simulink model "holo"  (R2012b)
settings: Solver=FixedStepDiscrete  SolverMode=SingleTasking  StartTime=0.0  StopTime=160000  RelTol=1e-3
undefined symbols (not defined in the file): xlipgetpartsetting
libraries: xbsIndex_r4 x3259, casper_library_misc x36, simulink x18, dspsigops x12, casper_library_delays x8, xps_library x5, casper_library_multipliers x4
(part 5 of 34)

== system holo/dec_fir1 ==
  sync_in : Inport
  real1 : Inport  Port=2
  imag1 : Inport  Port=3
  real2 : Inport  Port=4
  imag2 : Inport  Port=5
  real3 : Inport  Port=6
  imag3 : Inport  Port=7
  real4 : Inport  Port=8
  imag4 : Inport  Port=9
  convert1 : xbsIndex_r4/Convert  gui_display_data_type=Fixed-point  arith_type="Signed  (2's comp)"  n_bits=25  bin_pt=24  float_type=Single  exp_bits=8  fraction_bits=24  quantization="Round  (unbiased: +/- Inf)"  overflow=Wrap  en=off  latency=2  dbl_ovrd=off  pipeline=off  block_type=convert
  convert2 : xbsIndex_r4/Convert  gui_display_data_type=Fixed-point  arith_type="Signed  (2's comp)"  n_bits=25  bin_pt=24  float_type=Single  exp_bits=8  fraction_bits=24  quantization="Round  (unbiased: +/- Inf)"  overflow=Wrap  en=off  latency=2  dbl_ovrd=off  pipeline=off  block_type=convert
  delay : xbsIndex_r4/Delay  rst=off  infoeditControl=Selection of Reset will increase slice count due to use of real FFs and instead of SRLs  en=off  latency=7  dbl_ovrd=off  reg_retiming=off  block_type=delay
  fir_dbl_col1 : Subsystem  AncestorBlock=casper_library_downconverter/fir_dbl_col  mask(fir_dbl_col){n_inputs=4, coeff=[0.0082324    0.009013   0.0099508   -0.044769], add_latency=1, mult_latency=2, coeff_bit_width=18, coeff_bin_pt=17, first_stage_hdl=on, adder_imp=Behavioral}
      mask prompts: n_inputs "Inputs"; coeff "Coefficients"; add_latency "Add latency"; mult_latency "Mult Latency"; coeff_bit_width "Coefficient bit width"; coeff_bin_pt "Coefficient binary point"; first_stage_hdl "Implement first stage of adder trees on output as behavioural HDL"; adder_imp "Adder implementation"
      mask init: same as holo/dec_fir/fir_dbl_col1
      mask Help: eval('xlWeb(''http://casper.berkeley.edu/wiki/Fir_dbl_col'')')
      mask TypeOptions adder_imp: Behavioral | Fabric | DSP48
  fir_dbl_col10 : Subsystem  AncestorBlock=casper_library_downconverter/fir_dbl_col  mask(fir_dbl_col){n_inputs=4, coeff=[-0.0071276  -0.0069543  -0.0067009   -0.006375], add_latency=1, mult_latency=2, coeff_bit_width=18, coeff_bin_pt=17, first_stage_hdl=on, adder_imp=Behavioral}
      mask prompts: n_inputs "Inputs"; coeff "Coefficients"; add_latency "Add latency"; mult_latency "Mult Latency"; coeff_bit_width "Coefficient bit width"; coeff_bin_pt "Coefficient binary point"; first_stage_hdl "Implement first stage of adder trees on output as behavioural HDL"; adder_imp "Adder implementation"
      mask init: same as holo/dec_fir/fir_dbl_col1
      mask Help: eval('xlWeb(''http://casper.berkeley.edu/wiki/Fir_dbl_col'')')
      mask TypeOptions adder_imp: Behavioral | Fabric | DSP48
  fir_dbl_col11 : Subsystem  AncestorBlock=casper_library_downconverter/fir_dbl_col  mask(fir_dbl_col){n_inputs=4, coeff=[-0.0068894  -0.0071001  -0.0072066  -0.0072138], add_latency=1, mult_latency=2, coeff_bit_width=18, coeff_bin_pt=17, first_stage_hdl=on, adder_imp=Behavioral}
      mask prompts: n_inputs "Inputs"; coeff "Coefficients"; add_latency "Add latency"; mult_latency "Mult Latency"; coeff_bit_width "Coefficient bit width"; coeff_bin_pt "Coefficient binary point"; first_stage_hdl "Implement first stage of adder trees on output as behavioural HDL"; adder_imp "Adder implementation"
      mask init: same as holo/dec_fir/fir_dbl_col1
      mask Help: eval('xlWeb(''http://casper.berkeley.edu/wiki/Fir_dbl_col'')')
      mask TypeOptions adder_imp: Behavioral | Fabric | DSP48
  fir_dbl_col12 : Subsystem  AncestorBlock=casper_library_downconverter/fir_dbl_col  mask(fir_dbl_col){n_inputs=4, coeff=[-0.0049352  -0.0055949  -0.0061395  -0.0065702], add_latency=1, mult_latency=2, coeff_bit_width=18, coeff_bin_pt=17, first_stage_hdl=on, adder_imp=Behavioral}
      mask prompts: n_inputs "Inputs"; coeff "Coefficients"; add_latency "Add latency"; mult_latency "Mult Latency"; coeff_bit_width "Coefficient bit width"; coeff_bin_pt "Coefficient binary point"; first_stage_hdl "Implement first stage of adder trees on output as behavioural HDL"; adder_imp "Adder implementation"
      mask init: same as holo/dec_fir/fir_dbl_col1
      mask Help: eval('xlWeb(''http://casper.berkeley.edu/wiki/Fir_dbl_col'')')
      mask TypeOptions adder_imp: Behavioral | Fabric | DSP48
  fir_dbl_col13 : Subsystem  AncestorBlock=casper_library_downconverter/fir_dbl_col  mask(fir_dbl_col){n_inputs=4, coeff=[-0.0011588  -0.0022694  -0.0032709  -0.0041602], add_latency=1, mult_latency=2, coeff_bit_width=18, coeff_bin_pt=17, first_stage_hdl=on, adder_imp=Behavioral}
      mask prompts: n_inputs "Inputs"; coeff "Coefficients"; add_latency "Add latency"; mult_latency "Mult Latency"; coeff_bit_width "Coefficient bit width"; coeff_bin_pt "Coefficient binary point"; first_stage_hdl "Implement first stage of adder trees on output as behavioural HDL"; adder_imp "Adder implementation"
      mask init: same as holo/dec_fir/fir_dbl_col1
      mask Help: eval('xlWeb(''http://casper.berkeley.edu/wiki/Fir_dbl_col'')')
      mask TypeOptions adder_imp: Behavioral | Fabric | DSP48
  fir_dbl_col14 : Subsystem  AncestorBlock=casper_library_downconverter/fir_dbl_col  mask(fir_dbl_col){n_inputs=4, coeff=[0.0042713   0.0027787   0.0013712  5.6582e-05], add_latency=1, mult_latency=2, coeff_bit_width=18, coeff_bin_pt=17, first_stage_hdl=on, adder_imp=Behavioral}
      mask prompts: n_inputs "Inputs"; coeff "Coefficients"; add_latency "Add latency"; mult_latency "Mult Latency"; coeff_bit_width "Coefficient bit width"; coeff_bin_pt "Coefficient binary point"; first_stage_hdl "Implement first stage of adder trees on output as behavioural HDL"; adder_imp "Adder implementation"
      mask init: same as holo/dec_fir/fir_dbl_col1
      mask Help: eval('xlWeb(''http://casper.berkeley.edu/wiki/Fir_dbl_col'')')
      mask TypeOptions adder_imp: Behavioral | Fabric | DSP48
  fir_dbl_col15 : Subsystem  AncestorBlock=casper_library_downconverter/fir_dbl_col  mask(fir_dbl_col){n_inputs=4, coeff=[0.01091   0.0091708   0.0074773   0.0058407], add_latency=1, mult_latency=2, coeff_bit_width=18, coeff_bin_pt=17, first_stage_hdl=on, adder_imp=Behavioral}
      mask prompts: n_inputs "Inputs"; coeff "Coefficients"; add_latency "Add latency"; mult_latency "Mult Latency"; coeff_bit_width "Coefficient bit width"; coeff_bin_pt "Coefficient binary point"; first_stage_hdl "Implement first stage of adder trees on output as behavioural HDL"; adder_imp "Adder implementation"
      mask init: same as holo/dec_fir/fir_dbl_col1
      mask Help: eval('xlWeb(''http://casper.berkeley.edu/wiki/Fir_dbl_col'')')
      mask TypeOptions adder_imp: Behavioral | Fabric | DSP48
  fir_dbl_col16 : Subsystem  AncestorBlock=casper_library_downconverter/fir_dbl_col  mask(fir_dbl_col){n_inputs=4, coeff=[0.018084    0.016284    0.014479    0.012684], add_latency=1, mult_latency=2, coeff_bit_width=18, coeff_bin_pt=17, first_stage_hdl=on, adder_imp=Behavioral}
      mask prompts: n_inputs "Inputs"; coeff "Coefficients"; add_latency "Add latency"; mult_latency "Mult Latency"; coeff_bit_width "Coefficient bit width"; coeff_bin_pt "Coefficient binary point"; first_stage_hdl "Implement first stage of adder trees on output as behavioural HDL"; adder_imp "Adder implementation"
      mask init: same as holo/dec_fir/fir_dbl_col1
      mask Help: eval('xlWeb(''http://casper.berkeley.edu/wiki/Fir_dbl_col'')')
      mask TypeOptions adder_imp: Behavioral | Fabric | DSP48
  fir_dbl_col17 : Subsystem  AncestorBlock=casper_library_downconverter/fir_dbl_col  mask(fir_dbl_col){n_inputs=4, coeff=[0.02498    0.023329     0.02162    0.019867], add_latency=1, mult_latency=2, coeff_bit_width=18, coeff_bin_pt=17, first_stage_hdl=on, adder_imp=Behavioral}
      mask prompts: n_inputs "Inputs"; coeff "Coefficients"; add_latency "Add latency"; mult_latency "Mult Latency"; coeff_bit_width "Coefficient bit width"; coeff_bin_pt "Coefficient binary point"; first_stage_hdl "Implement first stage of adder trees on output as behavioural HDL"; adder_imp "Adder implementation"
      mask init: same as holo/dec_fir/fir_dbl_col1
      mask Help: eval('xlWeb(''http://casper.berkeley.edu/wiki/Fir_dbl_col'')')
      mask TypeOptions adder_imp: Behavioral | Fabric | DSP48
  fir_dbl_col18 : Subsystem  AncestorBlock=casper_library_downconverter/fir_dbl_col  mask(fir_dbl_col){n_inputs=4, coeff=[0.030764    0.029465    0.028061    0.026562], add_latency=1, mult_latency=2, coeff_bit_width=18, coeff_bin_pt=17, first_stage_hdl=on, adder_imp=Behavioral}
      mask prompts: n_inputs "Inputs"; coeff "Coefficients"; add_latency "Add latency"; mult_latency "Mult Latency"; coeff_bit_width "Coefficient bit width"; coeff_bin_pt "Coefficient binary point"; first_stage_hdl "Implement first stage of adder trees on output as behavioural HDL"; adder_imp "Adder implementation"
      mask init: same as holo/dec_fir/fir_dbl_col1
      mask Help: eval('xlWeb(''http://casper.berkeley.edu/wiki/Fir_dbl_col'')')
      mask TypeOptions adder_imp: Behavioral | Fabric | DSP48
  fir_dbl_col19 : Subsystem  AncestorBlock=casper_library_downconverter/fir_dbl_col  mask(fir_dbl_col){n_inputs=4, coeff=[0.034708    0.033927    0.033004    0.031947], add_latency=1, mult_latency=2, coeff_bit_width=18, coeff_bin_pt=17, first_stage_hdl=on, adder_imp=Behavioral}
      mask prompts: n_inputs "Inputs"; coeff "Coefficients"; add_latency "Add latency"; mult_latency "Mult Latency"; coeff_bit_width "Coefficient bit width"; coeff_bin_pt "Coefficient binary point"; first_stage_hdl "Implement first stage of adder trees on output as behavioural HDL"; adder_imp "Adder implementation"
      mask init: same as holo/dec_fir/fir_dbl_col1
      mask Help: eval('xlWeb(''http://casper.berkeley.edu/wiki/Fir_dbl_col'')')
      mask TypeOptions adder_imp: Behavioral | Fabric | DSP48
  fir_dbl_col2 : Subsystem  AncestorBlock=casper_library_downconverter/fir_dbl_col  mask(fir_dbl_col){n_inputs=4, coeff=[0.0062152   0.0065946   0.0070446   0.0075838], add_latency=1, mult_latency=2, coeff_bit_width=18, coeff_bin_pt=17, first_stage_hdl=on, adder_imp=Behavioral}
      mask prompts: n_inputs "Inputs"; coeff "Coefficients"; add_latency "Add latency"; mult_latency "Mult Latency"; coeff_bit_width "Coefficient bit width"; coeff_bin_pt "Coefficient binary point"; first_stage_hdl "Implement first stage of adder trees on output as behavioural HDL"; adder_imp "Adder implementation"
      mask init: same as holo/dec_fir/fir_dbl_col1
      mask Help: eval('xlWeb(''http://casper.berkeley.edu/wiki/Fir_dbl_col'')')
      mask TypeOptions adder_imp: Behavioral | Fabric | DSP48
  fir_dbl_col20 : Subsystem  AncestorBlock=casper_library_downconverter/fir_dbl_col  mask(fir_dbl_col){n_inputs=4, coeff=[0.036302    0.036141    0.035819     0.03534], add_latency=1, mult_latency=2, coeff_bit_width=18, coeff_bin_pt=17, first_stage_hdl=on, adder_imp=Behavioral}
      mask prompts: n_inputs "Inputs"; coeff "Coefficients"; add_latency "Add latency"; mult_latency "Mult Latency"; coeff_bit_width "Coefficient bit width"; coeff_bin_pt "Coefficient binary point"; first_stage_hdl "Implement first stage of adder trees on output as behavioural HDL"; adder_imp "Adder implementation"
      mask init: same as holo/dec_fir/fir_dbl_col1
      mask Help: eval('xlWeb(''http://casper.berkeley.edu/wiki/Fir_dbl_col'')')
      mask TypeOptions adder_imp: Behavioral | Fabric | DSP48
  fir_dbl_col3 : Subsystem  AncestorBlock=casper_library_downconverter/fir_dbl_col  mask(fir_dbl_col){n_inputs=4, coeff=[0.0051009   0.0053455   0.0056047   0.0058902], add_latency=1, mult_latency=2, coeff_bit_width=18, coeff_bin_pt=17, first_stage_hdl=on, adder_imp=Behavioral}
      mask prompts: n_inputs "Inputs"; coeff "Coefficients"; add_latency "Add latency"; mult_latency "Mult Latency"; coeff_bit_width "Coefficient bit width"; coeff_bin_pt "Coefficient binary point"; first_stage_hdl "Implement first stage of adder trees on output as behavioural HDL"; adder_imp "Adder implementation"
      mask init: same as holo/dec_fir/fir_dbl_col1
      mask Help: eval('xlWeb(''http://casper.berkeley.edu/wiki/Fir_dbl_col'')')
      mask TypeOptions adder_imp: Behavioral | Fabric | DSP48
  fir_dbl_col4 : Subsystem  AncestorBlock=casper_library_downconverter/fir_dbl_col  mask(fir_dbl_col){n_inputs=4, coeff=[0.0040818   0.0043581   0.0046155   0.0048606], add_latency=1, mult_latency=2, coeff_bit_width=18, coeff_bin_pt=17, first_stage_hdl=on, adder_imp=Behavioral}
      mask prompts: n_inputs "Inputs"; coeff "Coefficients"; add_latency "Add latency"; mult_latency "Mult Latency"; coeff_bit_width "Coefficient bit width"; coeff_bin_pt "Coefficient binary point"; first_stage_hdl "Implement first stage of adder trees on output as behavioural HDL"; adder_imp "Adder implementation"
      mask init: same as holo/dec_fir/fir_dbl_col1
      mask Help: eval('xlWeb(''http://casper.berkeley.edu/wiki/Fir_dbl_col'')')
      mask TypeOptions adder_imp: Behavioral | Fabric | DSP48
  fir_dbl_col5 : Subsystem  AncestorBlock=casper_library_downconverter/fir_dbl_col  mask(fir_dbl_col){n_inputs=4, coeff=[0.0026997   0.0030928   0.0034527   0.0037814], add_latency=1, mult_latency=2, coeff_bit_width=18, coeff_bin_pt=17, first_stage_hdl=on, adder_imp=Behavioral}
      mask prompts: n_inputs "Inputs"; coeff "Coefficients"; add_latency "Add latency"; mult_latency "Mult Latency"; coeff_bit_width "Coefficient bit width"; coeff_bin_pt "Coefficient binary point"; first_stage_hdl "Implement first stage of adder trees on output as behavioural HDL"; adder_imp "Adder implementation"
      mask init: same as holo/dec_fir/fir_dbl_col1
      mask Help: eval('xlWeb(''http://casper.berkeley.edu/wiki/Fir_dbl_col'')')
      mask TypeOptions adder_imp: Behavioral | Fabric | DSP48
  fir_dbl_col6 : Subsystem  AncestorBlock=casper_library_downconverter/fir_dbl_col  mask(fir_dbl_col){n_inputs=4, coeff=[0.00079599   0.0013192   0.0018123   0.0022728], add_latency=1, mult_latency=2, coeff_bit_width=18, coeff_bin_pt=17, first_stage_hdl=on, adder_imp=Behavioral}
      mask prompts: n_inputs "Inputs"; coeff "Coefficients"; add_latency "Add latency"; mult_latency "Mult Latency"; coeff_bit_width "Coefficient bit width"; coeff_bin_pt "Coefficient binary point"; first_stage_hdl "Implement first stage of adder trees on output as behavioural HDL"; adder_imp "Adder implementation"
      mask init: same as holo/dec_fir/fir_dbl_col1
      mask Help: eval('xlWeb(''http://casper.berkeley.edu/wiki/Fir_dbl_col'')')
      mask TypeOptions adder_imp: Behavioral | Fabric | DSP48
  fir_dbl_col7 : Subsystem  AncestorBlock=casper_library_downconverter/fir_dbl_col  mask(fir_dbl_col){n_inputs=4, coeff=[-0.0015248  -0.0009199 -0.00032795  0.00024561], add_latency=1, mult_latency=2, coeff_bit_width=18, coeff_bin_pt=17, first_stage_hdl=on, adder_imp=Behavioral}
      mask prompts: n_inputs "Inputs"; coeff "Coefficients"; add_latency "Add latency"; mult_latency "Mult Latency"; coeff_bit_width "Coefficient bit width"; coeff_bin_pt "Coefficient binary point"; first_stage_hdl "Implement first stage of adder trees on output as behavioural HDL"; adder_imp "Adder implementation"
      mask init: same as holo/dec_fir/fir_dbl_col1
      mask Help: eval('xlWeb(''http://casper.berkeley.edu/wiki/Fir_dbl_col'')')
      mask TypeOptions adder_imp: Behavioral | Fabric | DSP48
  fir_dbl_col8 : Subsystem  AncestorBlock=casper_library_downconverter/fir_dbl_col  mask(fir_dbl_col){n_inputs=4, coeff=[-0.0039413  -0.0033521  -0.0027479  -0.0021363], add_latency=1, mult_latency=2, coeff_bit_width=18, coeff_bin_pt=17, first_stage_hdl=on, adder_imp=Behavioral}
      mask prompts: n_inputs "Inputs"; coeff "Coefficients"; add_latency "Add latency"; mult_latency "Mult Latency"; coeff_bit_width "Coefficient bit width"; coeff_bin_pt "Coefficient binary point"; first_stage_hdl "Implement first stage of adder trees on output as behavioural HDL"; adder_imp "Adder implementation"
      mask init: same as holo/dec_fir/fir_dbl_col1
      mask Help: eval('xlWeb(''http://casper.berkeley.edu/wiki/Fir_dbl_col'')')
      mask TypeOptions adder_imp: Behavioral | Fabric | DSP48
  fir_dbl_col9 : Subsystem  AncestorBlock=casper_library_downconverter/fir_dbl_col  mask(fir_dbl_col){n_inputs=4, coeff=[-0.0059845  -0.0055375  -0.0050423  -0.0045074], add_latency=1, mult_latency=2, coeff_bit_width=18, coeff_bin_pt=17, first_stage_hdl=on, adder_imp=Behavioral}
      mask prompts: n_inputs "Inputs"; coeff "Coefficients"; add_latency "Add latency"; mult_latency "Mult Latency"; coeff_bit_width "Coefficient bit width"; coeff_bin_pt "Coefficient binary point"; first_stage_hdl "Implement first stage of adder trees on output as behavioural HDL"; adder_imp "Adder implementation"
      mask init: same as holo/dec_fir/fir_dbl_col1
      mask Help: eval('xlWeb(''http://casper.berkeley.edu/wiki/Fir_dbl_col'')')
      mask TypeOptions adder_imp: Behavioral | Fabric | DSP48
  imag_sum : Subsystem  AncestorBlock=casper_library_misc/adder_tree  mask(adder_tree){n_inputs=20, latency=1, adder_imp=Behavioral, first_stage_hdl=off}
      mask prompts: n_inputs "Number of Inputs"; latency "Add Latency"; adder_imp "Adder implementation"; first_stage_hdl "Use behavioural HDL for first stage of adders"
      mask help:
      | Sums all inputs using a tree of adds and delays.
      |
      | Number of inputs: The number of inputs to the block to be summed
      | Add latency: The number of clock cycles to perform one addition (affects timing)..
      | Adder implementation: choice of fabric or DSP48E core, or behavioral HDL
      | Use behavioural HDL for first stage of adders: Causes the first stage of adders to be absorbed into DSP blocks if multipliers precede them (Virtex 5). Overrides Adder implementation
      mask init:
      | adder_tree_init(gcb, ...
      |     'n_inputs', n_inputs, ...
      |     'latency', latency, ...
      |     'adder_imp', adder_imp, ...
      |     'first_stage_hdl', first_stage_hdl);
      settings: AttributesFormatString=latency 5
      mask Help: eval('xlWeb(''http://casper.berkeley.edu/wiki/Adder_tree'')')
      mask TypeOptions adder_imp: Behavioral | Fabric | DSP48
  real_sum : Subsystem  AncestorBlock=casper_library_misc/adder_tree  mask(adder_tree){n_inputs=20, latency=1, adder_imp=Behavioral, first_stage_hdl=off}
      mask prompts: n_inputs "Number of Inputs"; latency "Add Latency"; adder_imp "Adder implementation"; first_stage_hdl "Use behavioural HDL for first stage of adders"
      mask help:
      | Sums all inputs using a tree of adds and delays.
      |
      | Number of inputs: The number of inputs to the block to be summed
      | Add latency: The number of clock cycles to perform one addition (affects timing)..
      | Adder implementation: choice of fabric or DSP48E core, or behavioral HDL
      | Use behavioural HDL for first stage of adders: Causes the first stage of adders to be absorbed into DSP blocks if multipliers precede them (Virtex 5). Overrides Adder implementation
      mask init:
      | adder_tree_init(gcb, ...
      |     'n_inputs', n_inputs, ...
      |     'latency', latency, ...
      |     'adder_imp', adder_imp, ...
      |     'first_stage_hdl', first_stage_hdl);
      settings: AttributesFormatString=latency 5
      mask Help: eval('xlWeb(''http://casper.berkeley.edu/wiki/Adder_tree'')')
      mask TypeOptions adder_imp: Behavioral | Fabric | DSP48
  ri_to_c : casper_library_misc/ri_to_c
  shift1 : xbsIndex_r4/Shift  shift_dir=Left  shift_bits=1  en=off  latency=0  precision=Full  arith_type="Signed  (2's comp)"  n_bits=16  bin_pt=14  quantization=Truncate  overflow=Wrap  dbl_ovrd=off  block_type=shift
  shift2 : xbsIndex_r4/Shift  shift_dir=Left  shift_bits=1  en=off  latency=0  precision=Full  arith_type="Signed  (2's comp)"  n_bits=16  bin_pt=14  quantization=Truncate  overflow=Wrap  dbl_ovrd=off  block_type=shift
  sync_out : Outport
  dout : Outport  Port=2
  wires:
  real1/1 -> fir_dbl_col1/1(real1)
  imag1/1 -> fir_dbl_col1/2(imag1)
  real2/1 -> fir_dbl_col1/3(real2)
  imag2/1 -> fir_dbl_col1/4(imag2)
  real3/1 -> fir_dbl_col1/5(real3)
  imag3/1 -> fir_dbl_col1/6(imag3)
  real4/1 -> fir_dbl_col1/7(real4)
  imag4/1 -> fir_dbl_col1/8(imag4)
  fir_dbl_col1/17(real_sum) -> real_sum/2(din1)
  fir_dbl_col1/18(imag_sum) -> imag_sum/2(din1)
  fir_dbl_col1/1(real_out1) -> fir_dbl_col2/1(real1)
  fir_dbl_col1/2(imag_out1) -> fir_dbl_col2/2(imag1)
  fir_dbl_col1/3(real_out2) -> fir_dbl_col2/3(real2)
  fir_dbl_col1/4(imag_out2) -> fir_dbl_col2/4(imag2)
  fir_dbl_col1/5(real_out3) -> fir_dbl_col2/5(real3)
  fir_dbl_col1/6(imag_out3) -> fir_dbl_col2/6(imag3)
  fir_dbl_col1/7(real_out4) -> fir_dbl_col2/7(real4)
  fir_dbl_col1/8(imag_out4) -> fir_dbl_col2/8(imag4)
  fir_dbl_col2/17(real_sum) -> real_sum/3(din2)
  fir_dbl_col2/18(imag_sum) -> imag_sum/3(din2)
  fir_dbl_col2/1(real_out1) -> fir_dbl_col3/1(real1)
  fir_dbl_col2/2(imag_out1) -> fir_dbl_col3/2(imag1)
  fir_dbl_col2/3(real_out2) -> fir_dbl_col3/3(real2)
  fir_dbl_col2/4(imag_out2) -> fir_dbl_col3/4(imag2)
  fir_dbl_col2/5(real_out3) -> fir_dbl_col3/5(real3)
  fir_dbl_col2/6(imag_out3) -> fir_dbl_col3/6(imag3)
  fir_dbl_col2/7(real_out4) -> fir_dbl_col3/7(real4)
  fir_dbl_col2/8(imag_out4) -> fir_dbl_col3/8(imag4)
  fir_dbl_col3/17(real_sum) -> real_sum/4(din3)
  fir_dbl_col3/18(imag_sum) -> imag_sum/4(din3)
  fir_dbl_col3/1(real_out1) -> fir_dbl_col4/1(real1)
  fir_dbl_col3/2(imag_out1) -> fir_dbl_col4/2(imag1)
  fir_dbl_col3/3(real_out2) -> fir_dbl_col4/3(real2)
  fir_dbl_col3/4(imag_out2) -> fir_dbl_col4/4(imag2)
  fir_dbl_col3/5(real_out3) -> fir_dbl_col4/5(real3)
  fir_dbl_col3/6(imag_out3) -> fir_dbl_col4/6(imag3)
  fir_dbl_col3/7(real_out4) -> fir_dbl_col4/7(real4)
  fir_dbl_col3/8(imag_out4) -> fir_dbl_col4/8(imag4)
  fir_dbl_col4/17(real_sum) -> real_sum/5(din4)
  fir_dbl_col4/18(imag_sum) -> imag_sum/5(din4)
  fir_dbl_col4/1(real_out1) -> fir_dbl_col5/1(real1)
  fir_dbl_col4/2(imag_out1) -> fir_dbl_col5/2(imag1)
  fir_dbl_col4/3(real_out2) -> fir_dbl_col5/3(real2)
  fir_dbl_col4/4(imag_out2) -> fir_dbl_col5/4(imag2)
  fir_dbl_col4/5(real_out3) -> fir_dbl_col5/5(real3)
  fir_dbl_col4/6(imag_out3) -> fir_dbl_col5/6(imag3)
  fir_dbl_col4/7(real_out4) -> fir_dbl_col5/7(real4)
  fir_dbl_col4/8(imag_out4) -> fir_dbl_col5/8(imag4)
  fir_dbl_col5/17(real_sum) -> real_sum/6(din5)
  fir_dbl_col5/18(imag_sum) -> imag_sum/6(din5)
  fir_dbl_col5/1(real_out1) -> fir_dbl_col6/1(real1)
  fir_dbl_col5/2(imag_out1) -> fir_dbl_col6/2(imag1)
  fir_dbl_col5/3(real_out2) -> fir_dbl_col6/3(real2)
  fir_dbl_col5/4(imag_out2) -> fir_dbl_col6/4(imag2)
  fir_dbl_col5/5(real_out3) -> fir_dbl_col6/5(real3)
  fir_dbl_col5/6(imag_out3) -> fir_dbl_col6/6(imag3)
  fir_dbl_col5/7(real_out4) -> fir_dbl_col6/7(real4)
  fir_dbl_col5/8(imag_out4) -> fir_dbl_col6/8(imag4)
  fir_dbl_col6/17(real_sum) -> real_sum/7(din6)
  fir_dbl_col6/18(imag_sum) -> imag_sum/7(din6)
  fir_dbl_col6/1(real_out1) -> fir_dbl_col7/1(real1)
  fir_dbl_col6/2(imag_out1) -> fir_dbl_col7/2(imag1)
  fir_dbl_col6/3(real_out2) -> fir_dbl_col7/3(real2)
  fir_dbl_col6/4(imag_out2) -> fir_dbl_col7/4(imag2)
  fir_dbl_col6/5(real_out3) -> fir_dbl_col7/5(real3)
  fir_dbl_col6/6(imag_out3) -> fir_dbl_col7/6(imag3)
  fir_dbl_col6/7(real_out4) -> fir_dbl_col7/7(real4)
  fir_dbl_col6/8(imag_out4) -> fir_dbl_col7/8(imag4)
  fir_dbl_col7/17(real_sum) -> real_sum/8(din7)
  fir_dbl_col7/18(imag_sum) -> imag_sum/8(din7)
  fir_dbl_col7/1(real_out1) -> fir_dbl_col8/1(real1)
  fir_dbl_col7/2(imag_out1) -> fir_dbl_col8/2(imag1)
  fir_dbl_col7/3(real_out2) -> fir_dbl_col8/3(real2)
  fir_dbl_col7/4(imag_out2) -> fir_dbl_col8/4(imag2)
  fir_dbl_col7/5(real_out3) -> fir_dbl_col8/5(real3)
  fir_dbl_col7/6(imag_out3) -> fir_dbl_col8/6(imag3)
  fir_dbl_col7/7(real_out4) -> fir_dbl_col8/7(real4)
  fir_dbl_col7/8(imag_out4) -> fir_dbl_col8/8(imag4)
  fir_dbl_col8/17(real_sum) -> real_sum/9(din8)
  fir_dbl_col8/18(imag_sum) -> imag_sum/9(din8)
  fir_dbl_col8/1(real_out1) -> fir_dbl_col9/1(real1)
  fir_dbl_col8/2(imag_out1) -> fir_dbl_col9/2(imag1)
  fir_dbl_col8/3(real_out2) -> fir_dbl_col9/3(real2)
  fir_dbl_col8/4(imag_out2) -> fir_dbl_col9/4(imag2)
  fir_dbl_col8/5(real_out3) -> fir_dbl_col9/5(real3)
  fir_dbl_col8/6(imag_out3) -> fir_dbl_col9/6(imag3)
  fir_dbl_col8/7(real_out4) -> fir_dbl_col9/7(real4)
  fir_dbl_col8/8(imag_out4) -> fir_dbl_col9/8(imag4)
  fir_dbl_col9/17(real_sum) -> real_sum/10(din9)
  fir_dbl_col9/18(imag_sum) -> imag_sum/10(din9)
  fir_dbl_col9/1(real_out1) -> fir_dbl_col10/1(real1)
  fir_dbl_col9/2(imag_out1) -> fir_dbl_col10/2(imag1)
  fir_dbl_col9/3(real_out2) -> fir_dbl_col10/3(real2)
  fir_dbl_col9/4(imag_out2) -> fir_dbl_col10/4(imag2)
  fir_dbl_col9/5(real_out3) -> fir_dbl_col10/5(real3)
  fir_dbl_col9/6(imag_out3) -> fir_dbl_col10/6(imag3)
  fir_dbl_col9/7(real_out4) -> fir_dbl_col10/7(real4)
  fir_dbl_col9/8(imag_out4) -> fir_dbl_col10/8(imag4)
  fir_dbl_col10/17(real_sum) -> real_sum/11(din10)
  fir_dbl_col10/18(imag_sum) -> imag_sum/11(din10)
  fir_dbl_col10/1(real_out1) -> fir_dbl_col11/1(real1)
  fir_dbl_col10/2(imag_out1) -> fir_dbl_col11/2(imag1)
  fir_dbl_col10/3(real_out2) -> fir_dbl_col11/3(real2)
  fir_dbl_col10/4(imag_out2) -> fir_dbl_col11/4(imag2)
  fir_dbl_col10/5(real_out3) -> fir_dbl_col11/5(real3)
  fir_dbl_col10/6(imag_out3) -> fir_dbl_col11/6(imag3)
  fir_dbl_col10/7(real_out4) -> fir_dbl_col11/7(real4)
  fir_dbl_col10/8(imag_out4) -> fir_dbl_col11/8(imag4)
  fir_dbl_col11/17(real_sum) -> real_sum/12(din11)
  fir_dbl_col11/18(imag_sum) -> imag_sum/12(din11)
  fir_dbl_col11/1(real_out1) -> fir_dbl_col12/1(real1)
  fir_dbl_col11/2(imag_out1) -> fir_dbl_col12/2(imag1)
  fir_dbl_col11/3(real_out2) -> fir_dbl_col12/3(real2)
  fir_dbl_col11/4(imag_out2) -> fir_dbl_col12/4(imag2)
  fir_dbl_col11/5(real_out3) -> fir_dbl_col12/5(real3)
  fir_dbl_col11/6(imag_out3) -> fir_dbl_col12/6(imag3)
  fir_dbl_col11/7(real_out4) -> fir_dbl_col12/7(real4)
  fir_dbl_col11/8(imag_out4) -> fir_dbl_col12/8(imag4)
  fir_dbl_col12/17(real_sum) -> real_sum/13(din12)
  fir_dbl_col12/18(imag_sum) -> imag_sum/13(din12)
  fir_dbl_col12/1(real_out1) -> fir_dbl_col13/1(real1)
  fir_dbl_col12/2(imag_out1) -> fir_dbl_col13/2(imag1)
  fir_dbl_col12/3(real_out2) -> fir_dbl_col13/3(real2)
  fir_dbl_col12/4(imag_out2) -> fir_dbl_col13/4(imag2)
  fir_dbl_col12/5(real_out3) -> fir_dbl_col13/5(real3)
  fir_dbl_col12/6(imag_out3) -> fir_dbl_col13/6(imag3)
  fir_dbl_col12/7(real_out4) -> fir_dbl_col13/7(real4)
  fir_dbl_col12/8(imag_out4) -> fir_dbl_col13/8(imag4)
  fir_dbl_col13/17(real_sum) -> real_sum/14(din13)
  fir_dbl_col13/18(imag_sum) -> imag_sum/14(din13)
  fir_dbl_col13/1(real_out1) -> fir_dbl_col14/1(real1)
  fir_dbl_col13/2(imag_out1) -> fir_dbl_col14/2(imag1)
  fir_dbl_col13/3(real_out2) -> fir_dbl_col14/3(real2)
  fir_dbl_col13/4(imag_out2) -> fir_dbl_col14/4(imag2)
  fir_dbl_col13/5(real_out3) -> fir_dbl_col14/5(real3)
  fir_dbl_col13/6(imag_out3) -> fir_dbl_col14/6(imag3)
  fir_dbl_col13/7(real_out4) -> fir_dbl_col14/7(real4)
  fir_dbl_col13/8(imag_out4) -> fir_dbl_col14/8(imag4)
  fir_dbl_col14/17(real_sum) -> real_sum/15(din14)
  fir_dbl_col14/18(imag_sum) -> imag_sum/15(din14)
  fir_dbl_col14/1(real_out1) -> fir_dbl_col15/1(real1)
  fir_dbl_col14/2(imag_out1) -> fir_dbl_col15/2(imag1)
  fir_dbl_col14/3(real_out2) -> fir_dbl_col15/3(real2)
  fir_dbl_col14/4(imag_out2) -> fir_dbl_col15/4(imag2)
  fir_dbl_col14/5(real_out3) -> fir_dbl_col15/5(real3)
  fir_dbl_col14/6(imag_out3) -> fir_dbl_col15/6(imag3)
  fir_dbl_col14/7(real_out4) -> fir_dbl_col15/7(real4)
  fir_dbl_col14/8(imag_out4) -> fir_dbl_col15/8(imag4)
  fir_dbl_col15/17(real_sum) -> real_sum/16(din15)
  fir_dbl_col15/18(imag_sum) -> imag_sum/16(din15)
  fir_dbl_col15/1(real_out1) -> fir_dbl_col16/1(real1)
  fir_dbl_col15/2(imag_out1) -> fir_dbl_col16/2(imag1)
  fir_dbl_col15/3(real_out2) -> fir_dbl_col16/3(real2)
  fir_dbl_col15/4(imag_out2) -> fir_dbl_col16/4(imag2)
  fir_dbl_col15/5(real_out3) -> fir_dbl_col16/5(real3)
  fir_dbl_col15/6(imag_out3) -> fir_dbl_col16/6(imag3)
  fir_dbl_col15/7(real_out4) -> fir_dbl_col16/7(real4)
  fir_dbl_col15/8(imag_out4) -> fir_dbl_col16/8(imag4)
  fir_dbl_col16/17(real_sum) -> real_sum/17(din16)
  fir_dbl_col16/18(imag_sum) -> imag_sum/17(din16)
  fir_dbl_col16/1(real_out1) -> fir_dbl_col17/1(real1)
  fir_dbl_col16/2(imag_out1) -> fir_dbl_col17/2(imag1)
  fir_dbl_col16/3(real_out2) -> fir_dbl_col17/3(real2)
  fir_dbl_col16/4(imag_out2) -> fir_dbl_col17/4(imag2)
  fir_dbl_col16/5(real_out3) -> fir_dbl_col17/5(real3)
  fir_dbl_col16/6(imag_out3) -> fir_dbl_col17/6(imag3)
  fir_dbl_col16/7(real_out4) -> fir_dbl_col17/7(real4)
  fir_dbl_col16/8(imag_out4) -> fir_dbl_col17/8(imag4)
  fir_dbl_col17/17(real_sum) -> real_sum/18(din17)
  fir_dbl_col17/18(imag_sum) -> imag_sum/18(din17)
  fir_dbl_col17/1(real_out1) -> fir_dbl_col18/1(real1)
  fir_dbl_col17/2(imag_out1) -> fir_dbl_col18/2(imag1)
  fir_dbl_col17/3(real_out2) -> fir_dbl_col18/3(real2)
  fir_dbl_col17/4(imag_out2) -> fir_dbl_col18/4(imag2)
  fir_dbl_col17/5(real_out3) -> fir_dbl_col18/5(real3)
  fir_dbl_col17/6(imag_out3) -> fir_dbl_col18/6(imag3)
  fir_dbl_col17/7(real_out4) -> fir_dbl_col18/7(real4)
  fir_dbl_col17/8(imag_out4) -> fir_dbl_col18/8(imag4)
  fir_dbl_col18/17(real_sum) -> real_sum/19(din18)
  fir_dbl_col18/18(imag_sum) -> imag_sum/19(din18)
  fir_dbl_col18/1(real_out1) -> fir_dbl_col19/1(real1)
  fir_dbl_col18/2(imag_out1) -> fir_dbl_col19/2(imag1)
  fir_dbl_col18/3(real_out2) -> fir_dbl_col19/3(real2)
  fir_dbl_col18/4(imag_out2) -> fir_dbl_col19/4(imag2)
  fir_dbl_col18/5(real_out3) -> fir_dbl_col19/5(real3)
  fir_dbl_col18/6(imag_out3) -> fir_dbl_col19/6(imag3)
  fir_dbl_col18/7(real_out4) -> fir_dbl_col19/7(real4)
  fir_dbl_col18/8(imag_out4) -> fir_dbl_col19/8(imag4)
  fir_dbl_col19/17(real_sum) -> real_sum/20(din19)
  fir_dbl_col19/18(imag_sum) -> imag_sum/20(din19)
  fir_dbl_col19/1(real_out1) -> fir_dbl_col20/1(real1)
  fir_dbl_col19/2(imag_out1) -> fir_dbl_col20/2(imag1)
  fir_dbl_col19/3(real_out2) -> fir_dbl_col20/3(real2)
  fir_dbl_col19/4(imag_out2) -> fir_dbl_col20/4(imag2)
  fir_dbl_col19/5(real_out3) -> fir_dbl_col20/5(real3)
  fir_dbl_col19/6(imag_out3) -> fir_dbl_col20/6(imag3)
  fir_dbl_col19/7(real_out4) -> fir_dbl_col20/7(real4)
  fir_dbl_col19/8(imag_out4) -> fir_dbl_col20/8(imag4)
  fir_dbl_col20/17(real_sum) -> real_sum/21(din20)
  fir_dbl_col20/18(imag_sum) -> imag_sum/21(din20)
  real_sum/2(dout) -> shift1/1
  imag_sum/2(dout) -> shift2/1
  shift1/1 -> convert1/1
  shift2/1 -> convert2/1
  convert1/1 -> ri_to_c/1
  convert2/1 -> ri_to_c/2
  ri_to_c/1 -> dout/1
  sync_in/1 -> delay/1
  delay/1 -> real_sum/1(sync), imag_sum/1(sync)
  real_sum/1(sync_out) -> sync_out/1
  fir_dbl_col2/9(real_back_out1) -> fir_dbl_col1/9(real_back1)
  fir_dbl_col2/10(imag_back_out1) -> fir_dbl_col1/10(imag_back1)
  fir_dbl_col2/11(real_back_out2) -> fir_dbl_col1/11(real_back2)
  fir_dbl_col2/12(imag_back_out2) -> fir_dbl_col1/12(imag_back2)
  fir_dbl_col2/13(real_back_out3) -> fir_dbl_col1/13(real_back3)
  fir_dbl_col2/14(imag_back_out3) -> fir_dbl_col1/14(imag_back3)
  fir_dbl_col2/15(real_back_out4) -> fir_dbl_col1/15(real_back4)
  fir_dbl_col2/16(imag_back_out4) -> fir_dbl_col1/16(imag_back4)
  fir_dbl_col3/9(real_back_out1) -> fir_dbl_col2/9(real_back1)
  fir_dbl_col3/10(imag_back_out1) -> fir_dbl_col2/10(imag_back1)
  fir_dbl_col3/11(real_back_out2) -> fir_dbl_col2/11(real_back2)
  fir_dbl_col3/12(imag_back_out2) -> fir_dbl_col2/12(imag_back2)
  fir_dbl_col3/13(real_back_out3) -> fir_dbl_col2/13(real_back3)
  fir_dbl_col3/14(imag_back_out3) -> fir_dbl_col2/14(imag_back3)
  fir_dbl_col3/15(real_back_out4) -> fir_dbl_col2/15(real_back4)
  fir_dbl_col3/16(imag_back_out4) -> fir_dbl_col2/16(imag_back4)
  fir_dbl_col4/9(real_back_out1) -> fir_dbl_col3/9(real_back1)
  fir_dbl_col4/10(imag_back_out1) -> fir_dbl_col3/10(imag_back1)
  fir_dbl_col4/11(real_back_out2) -> fir_dbl_col3/11(real_back2)
  fir_dbl_col4/12(imag_back_out2) -> fir_dbl_col3/12(imag_back2)
  fir_dbl_col4/13(real_back_out3) -> fir_dbl_col3/13(real_back3)
  fir_dbl_col4/14(imag_back_out3) -> fir_dbl_col3/14(imag_back3)
  fir_dbl_col4/15(real_back_out4) -> fir_dbl_col3/15(real_back4)
  fir_dbl_col4/16(imag_back_out4) -> fir_dbl_col3/16(imag_back4)
  fir_dbl_col5/9(real_back_out1) -> fir_dbl_col4/9(real_back1)
  fir_dbl_col5/10(imag_back_out1) -> fir_dbl_col4/10(imag_back1)
  fir_dbl_col5/11(real_back_out2) -> fir_dbl_col4/11(real_back2)
  fir_dbl_col5/12(imag_back_out2) -> fir_dbl_col4/12(imag_back2)
  fir_dbl_col5/13(real_back_out3) -> fir_dbl_col4/13(real_back3)
  fir_dbl_col5/14(imag_back_out3) -> fir_dbl_col4/14(imag_back3)
  fir_dbl_col5/15(real_back_out4) -> fir_dbl_col4/15(real_back4)
  fir_dbl_col5/16(imag_back_out4) -> fir_dbl_col4/16(imag_back4)
  fir_dbl_col6/9(real_back_out1) -> fir_dbl_col5/9(real_back1)
  fir_dbl_col6/10(imag_back_out1) -> fir_dbl_col5/10(imag_back1)
  fir_dbl_col6/11(real_back_out2) -> fir_dbl_col5/11(real_back2)
  fir_dbl_col6/12(imag_back_out2) -> fir_dbl_col5/12(imag_back2)
  fir_dbl_col6/13(real_back_out3) -> fir_dbl_col5/13(real_back3)
  fir_dbl_col6/14(imag_back_out3) -> fir_dbl_col5/14(imag_back3)
  fir_dbl_col6/15(real_back_out4) -> fir_dbl_col5/15(real_back4)
  fir_dbl_col6/16(imag_back_out4) -> fir_dbl_col5/16(imag_back4)
  fir_dbl_col7/9(real_back_out1) -> fir_dbl_col6/9(real_back1)
  fir_dbl_col7/10(imag_back_out1) -> fir_dbl_col6/10(imag_back1)
  fir_dbl_col7/11(real_back_out2) -> fir_dbl_col6/11(real_back2)
  fir_dbl_col7/12(imag_back_out2) -> fir_dbl_col6/12(imag_back2)
  fir_dbl_col7/13(real_back_out3) -> fir_dbl_col6/13(real_back3)
  fir_dbl_col7/14(imag_back_out3) -> fir_dbl_col6/14(imag_back3)
  fir_dbl_col7/15(real_back_out4) -> fir_dbl_col6/15(real_back4)
  fir_dbl_col7/16(imag_back_out4) -> fir_dbl_col6/16(imag_back4)
  fir_dbl_col8/9(real_back_out1) -> fir_dbl_col7/9(real_back1)
  fir_dbl_col8/10(imag_back_out1) -> fir_dbl_col7/10(imag_back1)
  fir_dbl_col8/11(real_back_out2) -> fir_dbl_col7/11(real_back2)
  fir_dbl_col8/12(imag_back_out2) -> fir_dbl_col7/12(imag_back2)
  fir_dbl_col8/13(real_back_out3) -> fir_dbl_col7/13(real_back3)
  fir_dbl_col8/14(imag_back_out3) -> fir_dbl_col7/14(imag_back3)
  fir_dbl_col8/15(real_back_out4) -> fir_dbl_col7/15(real_back4)
  fir_dbl_col8/16(imag_back_out4) -> fir_dbl_col7/16(imag_back4)
  fir_dbl_col9/9(real_back_out1) -> fir_dbl_col8/9(real_back1)
  fir_dbl_col9/10(imag_back_out1) -> fir_dbl_col8/10(imag_back1)
  fir_dbl_col9/11(real_back_out2) -> fir_dbl_col8/11(real_back2)
  fir_dbl_col9/12(imag_back_out2) -> fir_dbl_col8/12(imag_back2)
  fir_dbl_col9/13(real_back_out3) -> fir_dbl_col8/13(real_back3)
  fir_dbl_col9/14(imag_back_out3) -> fir_dbl_col8/14(imag_back3)
  fir_dbl_col9/15(real_back_out4) -> fir_dbl_col8/15(real_back4)
  fir_dbl_col9/16(imag_back_out4) -> fir_dbl_col8/16(imag_back4)
  fir_dbl_col10/9(real_back_out1) -> fir_dbl_col9/9(real_back1)
  fir_dbl_col10/10(imag_back_out1) -> fir_dbl_col9/10(imag_back1)
  fir_dbl_col10/11(real_back_out2) -> fir_dbl_col9/11(real_back2)
  fir_dbl_col10/12(imag_back_out2) -> fir_dbl_col9/12(imag_back2)
  fir_dbl_col10/13(real_back_out3) -> fir_dbl_col9/13(real_back3)
  fir_dbl_col10/14(imag_back_out3) -> fir_dbl_col9/14(imag_back3)
  fir_dbl_col10/15(real_back_out4) -> fir_dbl_col9/15(real_back4)
  fir_dbl_col10/16(imag_back_out4) -> fir_dbl_col9/16(imag_back4)
  fir_dbl_col11/9(real_back_out1) -> fir_dbl_col10/9(real_back1)
  fir_dbl_col11/10(imag_back_out1) -> fir_dbl_col10/10(imag_back1)
  fir_dbl_col11/11(real_back_out2) -> fir_dbl_col10/11(real_back2)
  fir_dbl_col11/12(imag_back_out2) -> fir_dbl_col10/12(imag_back2)
  fir_dbl_col11/13(real_back_out3) -> fir_dbl_col10/13(real_back3)
  fir_dbl_col11/14(imag_back_out3) -> fir_dbl_col10/14(imag_back3)
  fir_dbl_col11/15(real_back_out4) -> fir_dbl_col10/15(real_back4)
  fir_dbl_col11/16(imag_back_out4) -> fir_dbl_col10/16(imag_back4)
  fir_dbl_col12/9(real_back_out1) -> fir_dbl_col11/9(real_back1)
  fir_dbl_col12/10(imag_back_out1) -> fir_dbl_col11/10(imag_back1)
  fir_dbl_col12/11(real_back_out2) -> fir_dbl_col11/11(real_back2)
  fir_dbl_col12/12(imag_back_out2) -> fir_dbl_col11/12(imag_back2)
  fir_dbl_col12/13(real_back_out3) -> fir_dbl_col11/13(real_back3)
  fir_dbl_col12/14(imag_back_out3) -> fir_dbl_col11/14(imag_back3)
  fir_dbl_col12/15(real_back_out4) -> fir_dbl_col11/15(real_back4)
  fir_dbl_col12/16(imag_back_out4) -> fir_dbl_col11/16(imag_back4)
  fir_dbl_col13/9(real_back_out1) -> fir_dbl_col12/9(real_back1)
  fir_dbl_col13/10(imag_back_out1) -> fir_dbl_col12/10(imag_back1)
  fir_dbl_col13/11(real_back_out2) -> fir_dbl_col12/11(real_back2)
  fir_dbl_col13/12(imag_back_out2) -> fir_dbl_col12/12(imag_back2)
  fir_dbl_col13/13(real_back_out3) -> fir_dbl_col12/13(real_back3)
  fir_dbl_col13/14(imag_back_out3) -> fir_dbl_col12/14(imag_back3)
  fir_dbl_col13/15(real_back_out4) -> fir_dbl_col12/15(real_back4)
  fir_dbl_col13/16(imag_back_out4) -> fir_dbl_col12/16(imag_back4)
  fir_dbl_col14/9(real_back_out1) -> fir_dbl_col13/9(real_back1)
  fir_dbl_col14/10(imag_back_out1) -> fir_dbl_col13/10(imag_back1)
  fir_dbl_col14/11(real_back_out2) -> fir_dbl_col13/11(real_back2)
  fir_dbl_col14/12(imag_back_out2) -> fir_dbl_col13/12(imag_back2)
  fir_dbl_col14/13(real_back_out3) -> fir_dbl_col13/13(real_back3)
  fir_dbl_col14/14(imag_back_out3) -> fir_dbl_col13/14(imag_back3)
  fir_dbl_col14/15(real_back_out4) -> fir_dbl_col13/15(real_back4)
  fir_dbl_col14/16(imag_back_out4) -> fir_dbl_col13/16(imag_back4)
  fir_dbl_col15/9(real_back_out1) -> fir_dbl_col14/9(real_back1)
  fir_dbl_col15/10(imag_back_out1) -> fir_dbl_col14/10(imag_back1)
  fir_dbl_col15/11(real_back_out2) -> fir_dbl_col14/11(real_back2)
  fir_dbl_col15/12(imag_back_out2) -> fir_dbl_col14/12(imag_back2)
  fir_dbl_col15/13(real_back_out3) -> fir_dbl_col14/13(real_back3)
  fir_dbl_col15/14(imag_back_out3) -> fir_dbl_col14/14(imag_back3)
  fir_dbl_col15/15(real_back_out4) -> fir_dbl_col14/15(real_back4)
  fir_dbl_col15/16(imag_back_out4) -> fir_dbl_col14/16(imag_back4)
  fir_dbl_col16/9(real_back_out1) -> fir_dbl_col15/9(real_back1)
  fir_dbl_col16/10(imag_back_out1) -> fir_dbl_col15/10(imag_back1)
  fir_dbl_col16/11(real_back_out2) -> fir_dbl_col15/11(real_back2)
  fir_dbl_col16/12(imag_back_out2) -> fir_dbl_col15/12(imag_back2)
  fir_dbl_col16/13(real_back_out3) -> fir_dbl_col15/13(real_back3)
  fir_dbl_col16/14(imag_back_out3) -> fir_dbl_col15/14(imag_back3)
  fir_dbl_col16/15(real_back_out4) -> fir_dbl_col15/15(real_back4)
  fir_dbl_col16/16(imag_back_out4) -> fir_dbl_col15/16(imag_back4)
  fir_dbl_col17/9(real_back_out1) -> fir_dbl_col16/9(real_back1)
  fir_dbl_col17/10(imag_back_out1) -> fir_dbl_col16/10(imag_back1)
  fir_dbl_col17/11(real_back_out2) -> fir_dbl_col16/11(real_back2)
  fir_dbl_col17/12(imag_back_out2) -> fir_dbl_col16/12(imag_back2)
  fir_dbl_col17/13(real_back_out3) -> fir_dbl_col16/13(real_back3)
  fir_dbl_col17/14(imag_back_out3) -> fir_dbl_col16/14(imag_back3)
  fir_dbl_col17/15(real_back_out4) -> fir_dbl_col16/15(real_back4)
  fir_dbl_col17/16(imag_back_out4) -> fir_dbl_col16/16(imag_back4)
  fir_dbl_col18/9(real_back_out1) -> fir_dbl_col17/9(real_back1)
  fir_dbl_col18/10(imag_back_out1) -> fir_dbl_col17/10(imag_back1)
  fir_dbl_col18/11(real_back_out2) -> fir_dbl_col17/11(real_back2)
  fir_dbl_col18/12(imag_back_out2) -> fir_dbl_col17/12(imag_back2)
  fir_dbl_col18/13(real_back_out3) -> fir_dbl_col17/13(real_back3)
  fir_dbl_col18/14(imag_back_out3) -> fir_dbl_col17/14(imag_back3)
  fir_dbl_col18/15(real_back_out4) -> fir_dbl_col17/15(real_back4)
  fir_dbl_col18/16(imag_back_out4) -> fir_dbl_col17/16(imag_back4)
  fir_dbl_col19/9(real_back_out1) -> fir_dbl_col18/9(real_back1)
  fir_dbl_col19/10(imag_back_out1) -> fir_dbl_col18/10(imag_back1)
  fir_dbl_col19/11(real_back_out2) -> fir_dbl_col18/11(real_back2)
  fir_dbl_col19/12(imag_back_out2) -> fir_dbl_col18/12(imag_back2)
  fir_dbl_col19/13(real_back_out3) -> fir_dbl_col18/13(real_back3)
  fir_dbl_col19/14(imag_back_out3) -> fir_dbl_col18/14(imag_back3)
  fir_dbl_col19/15(real_back_out4) -> fir_dbl_col18/15(real_back4)
  fir_dbl_col19/16(imag_back_out4) -> fir_dbl_col18/16(imag_back4)
  fir_dbl_col20/9(real_back_out1) -> fir_dbl_col19/9(real_back1)
  fir_dbl_col20/10(imag_back_out1) -> fir_dbl_col19/10(imag_back1)
  fir_dbl_col20/11(real_back_out2) -> fir_dbl_col19/11(real_back2)
  fir_dbl_col20/12(imag_back_out2) -> fir_dbl_col19/12(imag_back2)
  fir_dbl_col20/13(real_back_out3) -> fir_dbl_col19/13(real_back3)
  fir_dbl_col20/14(imag_back_out3) -> fir_dbl_col19/14(imag_back3)
  fir_dbl_col20/15(real_back_out4) -> fir_dbl_col19/15(real_back4)
  fir_dbl_col20/16(imag_back_out4) -> fir_dbl_col19/16(imag_back4)
  fir_dbl_col20/1(real_out1) -> fir_dbl_col20/9(real_back1)
  fir_dbl_col20/2(imag_out1) -> fir_dbl_col20/10(imag_back1)
  fir_dbl_col20/3(real_out2) -> fir_dbl_col20/11(real_back2)
  fir_dbl_col20/4(imag_out2) -> fir_dbl_col20/12(imag_back2)
  fir_dbl_col20/5(real_out3) -> fir_dbl_col20/13(real_back3)
  fir_dbl_col20/6(imag_out3) -> fir_dbl_col20/14(imag_back3)
  fir_dbl_col20/7(real_out4) -> fir_dbl_col20/15(real_back4)
  fir_dbl_col20/8(imag_out4) -> fir_dbl_col20/16(imag_back4)

== system holo/delay_wideband_prog0 ==
  sync : Inport
  delay : Inport  Port=2
  ld_delay : Inport  Port=3
  data_in0 : Inport  Port=4
  data_in1 : Inport  Port=5
  data_in2 : Inport  Port=6
  data_in3 : Inport  Port=7
  AddSub1 : xbsIndex_r4/AddSub  mode=Addition  use_carryin=off  use_carryout=off  en=off  latency=0  precision=Full  arith_type=Unsigned  n_bits=10  bin_pt=0  quantization=Truncate  overflow=Wrap  dbl_ovrd=off  use_behavioral_HDL=off  hw_selection=Fabric  pipelined=off  use_rpm=on  block_type=addsub
      settings: block_version=10.1.3
  AddSub2 : xbsIndex_r4/AddSub  mode=Addition  use_carryin=off  use_carryout=off  en=off  latency=0  precision=Full  arith_type=Unsigned  n_bits=10  bin_pt=0  quantization=Truncate  overflow=Wrap  dbl_ovrd=off  use_behavioral_HDL=off  hw_selection=Fabric  pipelined=off  use_rpm=on  block_type=addsub
      settings: block_version=10.1.3
  AddSub3 : xbsIndex_r4/AddSub  mode=Addition  use_carryin=off  use_carryout=off  en=off  latency=0  precision=Full  arith_type=Unsigned  n_bits=10  bin_pt=0  quantization=Truncate  overflow=Wrap  dbl_ovrd=off  use_behavioral_HDL=off  hw_selection=Fabric  pipelined=off  use_rpm=on  block_type=addsub
      settings: block_version=10.1.3
  Constant1 : xbsIndex_r4/Constant  const=2  gui_display_data_type=Fixed-point  arith_type=Unsigned  n_bits=2  bin_pt=0  preci_type=Single  exp_width=8  frac_width=24  explicit_period=on  period=1  equ=P=C  opselect=C  inp2=PCIN>>17  opr=+  inp1=P  carry=CIN  dbl_ovrd=off  block_type=constant
  Constant2 : xbsIndex_r4/Constant  const=1  gui_display_data_type=Fixed-point  arith_type=Unsigned  n_bits=2  bin_pt=0  preci_type=Single  exp_width=8  frac_width=24  explicit_period=on  period=1  equ=P=C  opselect=C  inp2=PCIN>>17  opr=+  inp1=P  carry=CIN  dbl_ovrd=off  block_type=constant
  Constant3 : xbsIndex_r4/Constant  const=0  gui_display_data_type=Fixed-point  arith_type=Unsigned  n_bits=2  bin_pt=0  preci_type=Single  exp_width=8  frac_width=24  explicit_period=on  period=1  equ=P=C  opselect=C  inp2=PCIN>>17  opr=+  inp1=P  carry=CIN  dbl_ovrd=off  block_type=constant
  Convert1 : xbsIndex_r4/Convert  gui_display_data_type=Fixed-point  arith_type=Unsigned  n_bits=1  bin_pt=0  float_type=Single  exp_bits=8  fraction_bits=24  quantization=Truncate  overflow=Wrap  en=off  latency=0  dbl_ovrd=off  pipeline=off  block_type=convert
      settings: block_version=10.1.3
  Convert2 : xbsIndex_r4/Convert  gui_display_data_type=Fixed-point  arith_type=Unsigned  n_bits=1  bin_pt=0  float_type=Single  exp_bits=8  fraction_bits=24  quantization=Truncate  overflow=Wrap  en=off  latency=0  dbl_ovrd=off  pipeline=off  block_type=convert
      settings: block_version=10.1.3
  Convert3 : xbsIndex_r4/Convert  gui_display_data_type=Fixed-point  arith_type=Unsigned  n_bits=1  bin_pt=0  float_type=Single  exp_bits=8  fraction_bits=24  quantization=Truncate  overflow=Wrap  en=off  latency=0  dbl_ovrd=off  pipeline=off  block_type=convert
      settings: block_version=10.1.3
  Relational1 : xbsIndex_r4/Relational  mode=a>b  en=off  latency=0  dbl_ovrd=off  block_type=relational
      settings: block_version=10.1.3
  Relational2 : xbsIndex_r4/Relational  mode=a>b  en=off  latency=0  dbl_ovrd=off  block_type=relational
      settings: block_version=10.1.3
  Relational3 : xbsIndex_r4/Relational  mode=a>b  en=off  latency=0  dbl_ovrd=off  block_type=relational
      settings: block_version=10.1.3
  barrel_switcher : Subsystem  AncestorBlock=casper_library_reorder/barrel_switcher  mask(barrel_switcher){n_inputs=2, async=off}
      mask prompts: n_inputs "Number of Inputs: (2^?)"; async "Asynchronous operation"
      mask help:
      | Shifts input to right by amount specified on sel,
      | wrapping around into higher order bits.
      mask init:
      | barrel_switcher_init(gcb,...
      |     'n_inputs', n_inputs, ...
      |     'async', async);
      mask Help: eval('xlWeb(''http://casper.berkeley.edu/wiki/Barrel_switcher'')')
  bram_rd_addrs : xbsIndex_r4/Slice  nbits=10  boolean_output=off  mode=Lower Bit Location + Width  bit1=0  base1=MSB of Input  bit0=2  base0=LSB of Input  dbl_ovrd=off  block_type=slice
      settings: infoedit="Extracts a given range of bits from each input sample and presents it at the output.  The output type is ordinarily unsigned with binary point at zero, but can be Boolean when the slice is one bit wide.<P><P>Hardware notes: In hardware this block costs nothing."  block_version=10.1.3
  delay_adder : xbsIndex_r4/AddSub  mode=Addition  use_carryin=off  use_carryout=off  en=off  latency=1  precision=Full  arith_type=Unsigned  n_bits=16  bin_pt=14  quantization=Truncate  overflow=Wrap  dbl_ovrd=off  use_behavioral_HDL=off  hw_selection=Fabric  pipelined=off  use_rpm=on  block_type=addsub
      settings: block_version=10.1.3
  delay_offset : xbsIndex_r4/Constant  const=12  gui_display_data_type=Fixed-point  arith_type=Unsigned  n_bits=12  bin_pt=0  preci_type=Single  exp_width=8  frac_width=24  explicit_period=on  period=1  equ=P=C  opselect=C  inp2=PCIN>>17  opr=+  inp1=P  carry=CIN  dbl_ovrd=off  block_type=constant
  delay_reg : xbsIndex_r4/Register  init=0  rst=off  en=on  dbl_ovrd=off  block_type=register
  delay_sel : xbsIndex_r4/Delay  rst=off  infoeditControl=Selection of Reset will increase slice count due to use of real FFs and instead of SRLs  en=off  latency=4  dbl_ovrd=off  reg_retiming=on  block_type=delay
  delay_sp{0..3} (4 alike) : casper_library_delays/delay_bram_prog  MaxDelay=10  bram_latency=2
  max_delay : xbsIndex_r4/Constant  const=4083  gui_display_data_type=Fixed-point  arith_type=Unsigned  n_bits=12  bin_pt=0  preci_type=Single  exp_width=8  frac_width=24  explicit_period=on  period=1  equ=P=C  opselect=C  inp2=PCIN>>17  opr=+  inp1=P  carry=CIN  dbl_ovrd=off  block_type=constant
  max_delay_chk : xbsIndex_r4/Relational  mode=a<=b  en=off  latency=1  dbl_ovrd=off  block_type=relational
      settings: block_version=10.1.3
  mux_delay : xbsIndex_r4/Mux  inputs=2  en=off  latency=0  precision=Full  arith_type=Unsigned  n_bits=16  bin_pt=14  quantization=Truncate  overflow=Wrap  dbl_ovrd=off  block_type=mux
  shift_sel : xbsIndex_r4/Slice  nbits=2  boolean_output=off  mode=Lower Bit Location + Width  bit1=0  base1=MSB of Input  bit0=0  base0=LSB of Input  dbl_ovrd=off  block_type=slice
  sync_delay : xbsIndex_r4/Delay  rst=off  infoeditControl=Selection of Reset will increase slice count due to use of real FFs and instead of SRLs  en=off  latency=16  dbl_ovrd=off  reg_retiming=on  block_type=delay
  sync_out : Outport
  data_out0 : Outport  Port=2
  data_out1 : Outport  Port=3
  data_out2 : Outport  Port=4
  data_out3 : Outport  Port=5
  wires:
  sync/1 -> sync_delay/1
  delay/1 -> delay_reg/1
  ld_delay/1 -> delay_reg/2
  delay_offset/1 -> delay_adder/2
  delay_adder/1 -> bram_rd_addrs/1, shift_sel/1
  delay_reg/1 -> max_delay_chk/1, mux_delay/3
  max_delay/1 -> max_delay_chk/2, mux_delay/2
  mux_delay/1 -> delay_adder/1
  max_delay_chk/1 -> mux_delay/1
  sync_delay/1 -> barrel_switcher/2(sync_in)
  barrel_switcher/1(sync_out) -> sync_out/1
  shift_sel/1 -> delay_sel/1, Relational1/1, Relational2/1, Relational3/1
  delay_sel/1 -> barrel_switcher/1(sel)
  barrel_switcher/5(Out4) -> data_out0/1
  barrel_switcher/4(Out3) -> data_out1/1
  barrel_switcher/3(Out2) -> data_out2/1
  barrel_switcher/2(Out1) -> data_out3/1
  data_in0/1 -> delay_sp0/1
  delay_sp0/1 -> barrel_switcher/6(In4)
  bram_rd_addrs/1 -> delay_sp0/2, AddSub1/1, AddSub2/1, AddSub3/1
  data_in1/1 -> delay_sp1/1
  delay_sp1/1 -> barrel_switcher/5(In3)
  Constant1/1 -> Relational1/2
  Relational1/1 -> Convert1/1
  Convert1/1 -> AddSub1/2
  AddSub1/1 -> delay_sp1/2
  data_in2/1 -> delay_sp2/1
  delay_sp2/1 -> barrel_switcher/4(In2)
  Constant2/1 -> Relational2/2
  Relational2/1 -> Convert2/1
  Convert2/1 -> AddSub2/2
  AddSub2/1 -> delay_sp2/2
  data_in3/1 -> delay_sp3/1
  delay_sp3/1 -> barrel_switcher/3(In1)
  Constant3/1 -> Relational3/2
  Relational3/1 -> Convert3/1
  Convert3/1 -> AddSub3/2
  AddSub3/1 -> delay_sp3/2
